simulink model "Parbtest"  (R2013a)
settings: Solver=VariableStepDiscrete  StartTime=0.0  StopTime=1  RelTol=1e-3
settings Model: Creator=dcollins3  LastModifiedBy=dcollins3

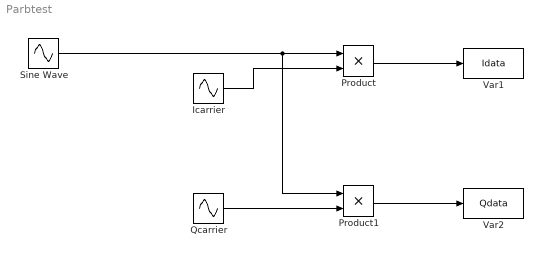
== system Parbtest ==
  Icarrier : Sin  Frequency=2*pi*100  Phase=-pi/2  Samples=519  SampleTime=inv(399)
  Product : Product
  Product1 : Product
  Qcarrier : Sin  Frequency=2*pi*100  Samples=519  SampleTime=inv(399)
  Sine Wave : Sin  Amplitude=3  Frequency=2*pi*1  Samples=52e3-1  SampleTime=inv(399)
  Var1 : ToWorkspace  VariableName=Idata  SampleTime=-1  SaveFormat=Timeseries
  Var2 : ToWorkspace  VariableName=Qdata  SampleTime=-1  SaveFormat=Timeseries
  wires:
  Sine Wave/1 -> Product1/1, Product/1
  Icarrier/1 -> Product/2
  Qcarrier/1 -> Product1/2
  Product/1 -> Var1/1
  Product1/1 -> Var2/1
